simulink model "sgMdl_IO334_AnalogLoopbackOversampling"  (R2024b)
settings: Solver=FixedStepAuto  StartTime=0.0  StopTime=inf  RelTol=1e-3
undefined symbols (not defined in the file): AnalogOutputFrameSize, IO3xx, Pull, pull, SineFrequency, Ts, up
libraries: speedgoatlib_fpga_analog_io x3, slrealtimeloglib x2, simulink x1, speedgoatlib_interrupt x1, slrealtimetgmanagement x1, speedgoatlib_fpga x1
Description:
  | IO334 - Analog Loopback with Oversampling
settings Model: ModifiedByFormat=Speedgoat  SimulationMode=external  ExtModeTrigDuration=100000  Creator=Speedgoat  LastModifiedBy=Speedgoat
settings SolverCC: ConcurrentTasks=on  PositivePriorityOrder=on
settings DataIOCC: SaveFormat=StructureWithTime
settings OptimizationCC: BlockReduction=off  OptimizeBlockIOStorage=off  BufferReuse=off  ReuseModelBlockBuffer=off
settings DebuggingCC: UnderspecifiedInitializationDetection=Classic  MergeDetectMultiDrivingBlocksExec=none  TasksWithSamePriorityMsg=none
settings HardwareCC: ProdBitPerLong=64  ProdLongLongMode=on  ProdHWDeviceType=Intel->x86-64 (Linux 64)
settings ModelReferenceCC: EnableRefExpFcnMdlSchedulingChecks=on  PropagateSignalLabelsOutOfModel=off
settings RTWCC: Description=Speedgoat Real-Time Target Machine  SystemTargetFile=speedgoat.tlc  TemplateMakefile=slrealtime_default_tmf  PostCodeGenCommand=sg.model.build.makeCfg(bdroot, buildInfo);  Toolchain=Simulink Real-Time Toolchain  BuildConfiguration=Faster Runs  TargetLang=C++  GPUComputeCapability=3.5
settings SimulinkRealTimeTargetCC: SubcomponentCodeInterfacePackaging=Reusable function  InstructionSetFMA=off  LogToMDFFile=off  SLRTFileLogMaxRuns=10
settings ConfigComp: CovBoundaryAbsTol=1.0e-5

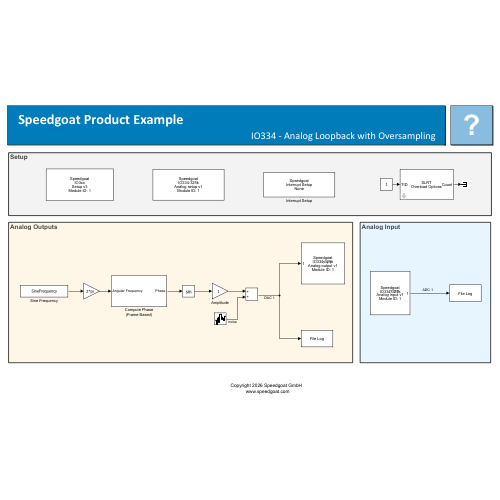
[thumbnail: Simulink's stored preview of the top-level diagram]
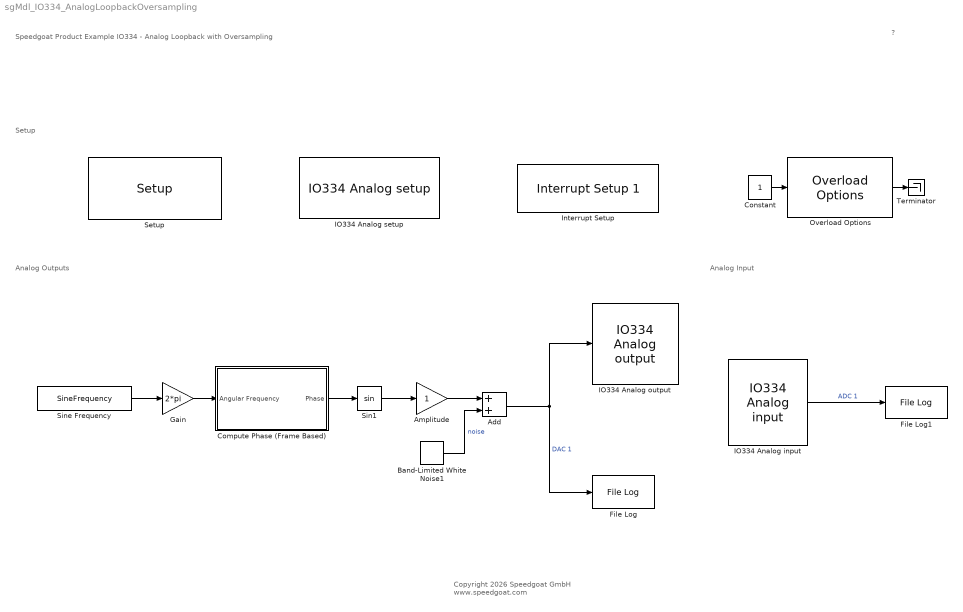
== system sgMdl_IO334_AnalogLoopbackOversampling ==
  note: Analog Outputs
  note: Analog Input
  note: Setup
  note: Speedgoat Product Example
      | IO334 - Analog Loopback with Oversampling
  note: ?
  note: Copyright 2026 Speedgoat GmbH
      |  www.speedgoat.com
  Add : Sum
  Amplitude : Gain
  Band-Limited White Noise1 : simulink/Sources/Band-Limited White Noise  Cov=[1e-6]  Ts=Ts  seed=round(rand(1,AnalogOutputFrameSize)*1000)
  Compute Phase (Frame Based) : Subsystem
  Constant : Constant  SampleTime=Ts
  File Log : slrealtimeloglib/File Log  decimation=1  inputProcessing=Columns as channels (frame based)
  File Log1 : slrealtimeloglib/File Log  decimation=1  inputProcessing=Elements as channels (sample based)
  Gain : Gain  Gain=2*pi
  IO334 Analog input : speedgoatlib_fpga_analog_io/IO334/IO334 Analog input  id=1  parSampleTime=-1  pciSlot=[-1,-1]  parAiChannels=1  parAiChannelsStreamed=1  parAiReadPrevValue=0  parAiEnableFrame=0  parAdcCoupling=[1 1 1 1]  parAdcContSampling=0  parAdcDmaEnable=0  parAdcActiveDmaDevices=[1 1 1 1]  parAiFrameSize=100
      settings: SourceProductName=Analog IO
  IO334 Analog output : speedgoatlib_fpga_analog_io/IO334/IO334 Analog output  id=1  parSampleTime=-1  pciSlot=[-1,-1]  board=Please select...  parAoChannels=1  parAoVoltageRange=1  parDacOverRange=[0 0 0 0 0 0 0 0]  parAoInitValues=0  parAoReset=0  parDacSyncOut=1  parAoEnableFrame=1  parDacActiveDmaDevices=[1 1 1 1]  parDacDmaLatency=2  parAoFrameSize=100
      settings: SourceProductName=Analog IO
  IO334 Analog setup : speedgoatlib_fpga_analog_io/IO334/IO334 Analog setup  id=1  parEnableCodeModule1=off  parEnableCodeModule2=off  parEnableCodeModule3=off  parEnableCodeModule4=off  parEnableCodeModule5=off  parEnableCodeModule6=off  parEnableCodeModule7=off  parEnableCodeModule8=off  parAdcEnableIndividualTrigger=off  parAdcDisableSampleRead=off  parAdcTriggerMode1=I/O Module Digital I/O  parAdcSampleRate1=1e6  parAdcDioTriggerChannel1=1  parAdcInternalTrigger1=<empty>  parAdcOversampling1=4  parAdcTriggerMode2=Model Step  parAdcSampleRate2=1e6  parAdcDioTriggerChannel2=1  parAdcInternalTrigger2=<empty>  parAdcOversampling2=4  parAdcTriggerMode3=I/O Module Digital I/O  parAdcSampleRate3=1e6  parAdcDioTriggerChannel3=1  parAdcInternalTrigger3=<empty>  parAdcOversampling3=4  parAdcTriggerMode4=I/O Module Internal Signal  parAdcSampleRate4=1e6  parAdcDioTriggerChannel4=1  parAdcInternalTrigger4=<empty>  parAdcOversampling4=4  parAdcTriggerMode5=I/O Module Clock  parAdcSampleRate5=1e6  parAdcDioTriggerChannel5=1  parAdcInternalTrigger5=<empty>  parAdcOversampling5=4  parAdcTriggerMode6=I/O Module Clock  parAdcSampleRate6=1e6  parAdcDioTriggerChannel6=1  parAdcInternalTrigger6=<empty>  parAdcOversampling6=4  parAdcTriggerMode7=I/O Module Clock  parAdcSampleRate7=1e6  parAdcDioTriggerChannel7=1  parAdcInternalTrigger7=<empty>  parAdcOversampling7=4  parAdcTriggerMode8=I/O Module Clock  parAdcSampleRate8=1e6  parAdcDioTriggerChannel8=1  parAdcInternalTrigger8=<empty>  parAdcOversampling8=4  parAdcReadPrevValueIndividualTrigger=off  parAdcEnableFrame=off  parAdcTriggerMode=I/O Module Clock  parAdcReadPrevValue=on  parAdcSampleRate=AnalogInputSampleRate  parAdcDioTriggerChannel=1  parAdcInternalTrigger=<empty>  parAdcOversampling=64  parAdcTriggerResolution=1e-08  parAdcSampleRateFrame=-1  parAdcFrameSize=100  parAdcSampleTime=Ts  parDacTriggerMode=I/O Module Clock  parDacInternalTrigger=<empty>  parDacDioTriggerChannel=1  parDacEnableFrame=on  dacUsesTimer=off  parDacFifoThreshold=AnalogOutputFrameSize*0.2  parDacTriggerResolution=1e-08  parDacSampleRate=-1  parDacFrameSize=AnalogOutputFrameSize  parDacSampleTime=Ts  parAdcChannel1=on  parAdcChannel2=off  parAdcChannel3=off  parAdcChannel4=off  parAdcChannel5=off  parAdcChannel6=off  parAdcChannel7=off  parAdcChannel8=off  parAdcChannel9=off  parAdcChannel10=off  parAdcChannel11=off  parAdcChannel12=off  parAdcChannel13=off  parAdcChannel14=off  parAdcChannel15=off  parAdcChannel16=off  parAdcAutoCorrection=on  parDacChannel1=on  parDacChannel2=off  parDacChannel3=off  parDacChannel4=off  parDacChannel5=off  parDacChannel6=off  parDacChannel7=off  parDacChannel8=off  parDacChannel9=off  parDacChannel10=off  parDacChannel11=off  parDacChannel12=off  parDacChannel13=off  parDacChannel14=off  parDacChannel15=off  parDacChannel16=off  parDacRange1=+-10 V  parDacInitValue1=0  parDacReset1=off  parDacRange2=+-5 V  parDacInitValue2=0  parDacReset2=off  parDacRange3=+-5 V  parDacInitValue3=0  parDacReset3=off  parDacRange4=+-5 V  parDacInitValue4=0  parDacReset4=off  parDacRange5=+-5 V  parDacInitValue5=0  parDacReset5=off  parDacRange6=+-5 V  parDacInitValue6=0  parDacReset6=off  parDacRange7=+-5 V  parDacInitValue7=0  parDacReset7=off  parDacRange8=+-5 V  parDacInitValue8=0  parDacReset8=off  parDacRange9=+-5 V  parDacInitValue9=0  parDacReset9=off  parDacRange10=+-5 V  parDacInitValue10=0  parDacReset10=off  parDacRange11=+-5 V  parDacInitValue11=0  parDacReset11=off  parDacRange12=+-5 V  parDacInitValue12=0  parDacReset12=off  parDacRange13=+-5 V  parDacInitValue13=0  parDacReset13=off  parDacRange14=+-5 V  parDacInitValue14=0  parDacReset14=off  parDacRange15=+-5 V  parDacInitValue15=0  parDacReset15=off  parDacRange16=+-5 V  parDacInitValue16=0  parDacReset16=off  parDacAutoCorrection=on
      settings: SourceProductName=Analog IO
  Interrupt Setup : speedgoatlib_interrupt/Interrupt Setup 1  parModuleTrigger=on  parPollingMode=on  parPriorityConf=High  parPriority=98  confStartFcn=IO334_325k_ANALOG_OUT_start_public  confStopFcn=IO334_325k_ANALOG_OUT_stop_public  confIsrFcn=IO334_325k_ANALOG_OUT_isr_public  confMapFcn=IO334_325k_ANALOG_OUT_map_public  confHookFile=io334_325k_analog_out_int_hooks.c  confIrqNr=-1  confIsPolling=on  confModID=16776961  confSelectedInt=Speedgoat IO334-325k Analog output interrupt  confSelectedId=1  confSelectedChannel=[]  confData=[90 1]  confForcePollingMode=off
  Overload Options : slrealtimetgmanagement/Overload Options  startupDur=1  startupDurSrc=Tunable Parameter  maxOverload=1  maxOverloadSrc=Tunable Parameter  TETFlag=off
  Setup : speedgoatlib_fpga/Setup/Setup  board=Please select...  id=1  pciSlot=-1  device_id=1  bitstreamFilePath=C:\SVN\speedgoatlib\releases\10.0.0\product_examples\IO334  bitstreamFile=Please select...  fpgaFreq=[100000000 125000000]  enableDma=on  rearEnb_1=off  rearIO_1=IO3xx-21  rearEnb_2=off  rearIO_2=None  ProgSpiFlash=off  ProgBPIFlash=off  useFpgaDmaController=off  dmaTrigDropdown=Model Step  dmaTrigSelect=0  dmaStopOnOverload=on  dmaModeSequential=on  dmaModeParallel=off  PullRPort15=pull-up 3.3V  PullRPort31=pull-up 3.3V  PullRPort47=pull-up 3.3V  PullRPort63=pull-up 3.3V  diffLineTermination_1=on  diffLineTermination_2=on  diffLineTermination_3=on  diffLineTermination_4=on  diffLineTermination_5=on  diffLineTermination_6=on  diffLineTermination_7=on  diffLineTermination_8=on  diffLineTermination_9=on  diffLineTermination_10=on  diffLineTermination_11=on  diffLineTermination_12=on  diffLineTermination_13=on  diffLineTermination_14=on  diffLineTermination_15=on  diffLineTermination_16=on  diffLineTermination_17=on  diffLineTermination_18=on  diffLineTermination_19=on  diffLineTermination_20=on  diffLineTermination_21=on  diffLineTermination_22=on  diffLineTermination_23=on  diffLineTermination_24=on  diffLineTermination_25=on  diffLineTermination_26=on  diffLineTermination_27=on  diffLineTermination_28=on  diffLineTermination_29=on  diffLineTermination_30=on  diffLineTermination_31=on  diffLineTermination_32=on  ioVoltageDropDown1=3.3V  pullResistorDropDown1_1=Pull-up  pullResistorDropDown1_2=Pull-up  pullResistorDropDown1_3=Pull-up  pullResistorDropDown1_4=Pull-up  pullResistorDropDown1_5=Pull-up  pullResistorDropDown1_6=Pull-up  pullResistorDropDown1_7=Pull-up  pullResistorDropDown1_8=Pull-up  ttlIsImplementedCheckBox1=off  pullResistorDropDown2=Pull-up  ioVoltageDropDown2=3.3V  ttlIsImplementedCheckBox2=off  pullResistorDropDown3=Pull-up  ioVoltageDropDown3=3.3V  ttlIsImplementedCheckBox3=off  pullResistorDropDown4=Pull-up  ioVoltageDropDown4=3.3V  ttlIsImplementedCheckBox4=off  pullResistorDropDown5=Pull-up  ioVoltageDropDown5=3.3V  ttlIsImplementedCheckBox5=off  pullResistorDropDown6=Pull-up  ioVoltageDropDown6=3.3V  ttlIsImplementedCheckBox6=off  pullResistorDropDown7=Pull-up  ioVoltageDropDown7=3.3V  ttlIsImplementedCheckBox7=off  pullResistorDropDown8=Pull-up  ioVoltageDropDown8=3.3V  ttlIsImplementedCheckBox8=off  terminationCheckBox1=off  terminationCheckBox2=off  terminationCheckBox3=off  terminationCheckBox4=off  diffIsImplementedCheckBox1=off  terminationCheckBox5=off  terminationCheckBox6=off  terminationCheckBox7=off  terminationCheckBox8=off  diffIsImplementedCheckBox2=off  terminationCheckBox9=off  terminationCheckBox10=off  terminationCheckBox11=off  terminationCheckBox12=off  diffIsImplementedCheckBox3=off  terminationCheckBox13=off  terminationCheckBox14=off  terminationCheckBox15=off  terminationCheckBox16=off  diffIsImplementedCheckBox4=off  terminationCheckBox17=off  terminationCheckBox18=off  terminationCheckBox19=off  terminationCheckBox20=off  diffIsImplementedCheckBox5=off  terminationCheckBox21=off  terminationCheckBox22=off  terminationCheckBox23=off  terminationCheckBox24=off  diffIsImplementedCheckBox6=off  terminationCheckBox25=off  terminationCheckBox26=off  terminationCheckBox27=off  terminationCheckBox28=off  diffIsImplementedCheckBox7=off  terminationCheckBox29=off  terminationCheckBox30=off  terminationCheckBox31=off  terminationCheckBox32=off  diffIsImplementedCheckBox8=off  PullRPort0_1=pull-up  VioPort0_1=3.3V  PullRPort1_1=pull-up  VioPort1_1=3.3V  PullRPort2_1=pull-up  VioPort2_1=3.3V  PullRPort3_1=pull-up  VioPort3_1=3.3V  PullRPort4_1=pull-up  VioPort4_1=3.3V  PullRPort5_1=pull-up  VioPort5_1=3.3V  PullRPort6_1=pull-up  VioPort6_1=3.3V  diffLineTermination_rear1_1=on  diffLineTermination_rear1_2=on  diffLineTermination_rear1_3=on  diffLineTermination_rear1_4=on  diffLineTermination_rear1_5=on  diffLineTermination_rear1_6=on  diffLineTermination_rear1_7=on  diffLineTermination_rear1_8=on  PullRPort0_2=pull-up  VioPort0_2=3.3V  PullRPort1_2=pull-up  VioPort1_2=3.3V  PullRPort2_2=pull-up  VioPort2_2=3.3V  PullRPort3_2=pull-up  VioPort3_2=3.3V  PullRPort4_2=pull-up  VioPort4_2=3.3V  PullRPort5_2=pull-up  VioPort5_2=3.3V  PullRPort6_2=pull-up  VioPort6_2=3.3V  diffLineTermination_rear2_1=on  diffLineTermination_rear2_2=on  diffLineTermination_rear2_3=on  diffLineTermination_rear2_4=on  diffLineTermination_rear2_5=on  diffLineTermination_rear2_6=on  diffLineTermination_rear2_7=on  diffLineTermination_rear2_8=on
      settings: SourceProductName=IO3xx
  Sin1 : Trigonometry
  Sine Frequency : Constant  Value=SineFrequency  SampleTime=Ts
  Terminator : Terminator
  wires:
  IO334 Analog input/1 -> File Log1/1  "ADC 1"
  Overload Options/1 -> Terminator/1
  Constant/1 -> Overload Options/1
  Gain/1 -> Compute Phase (Frame Based)/1(Angular Frequency)
  Sin1/1 -> Amplitude/1
  Amplitude/1 -> Add/1
  Add/1 -> IO334 Analog output/1, File Log/1  "DAC 1"
  Compute Phase (Frame Based)/1(Phase) -> Sin1/1
  Band-Limited White Noise1/1 -> Add/2  "noise"
  Sine Frequency/1 -> Gain/1

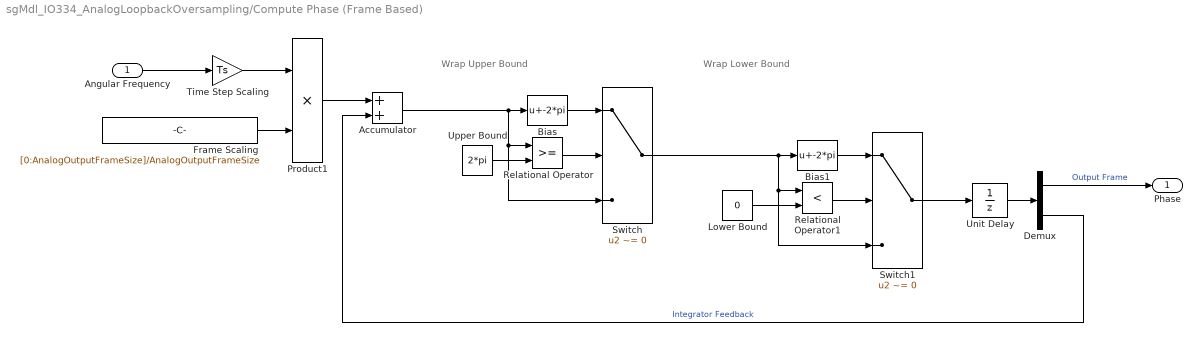
== system sgMdl_IO334_AnalogLoopbackOversampling/Compute Phase (Frame Based) ==
  note: Wrap Upper Bound
  note: Wrap Lower Bound
  Angular Frequency : Inport
  Accumulator : Sum
  Bias : Bias  Bias=-2*pi  SaturateOnIntegerOverflow=off
  Bias1 : Bias  Bias=-2*pi  SaturateOnIntegerOverflow=off
  Demux : Demux  Outputs=[AnalogOutputFrameSize,1]
  Frame Scaling : Constant  Value=[0:AnalogOutputFrameSize]/AnalogOutputFrameSize
  Lower Bound : Constant  Value=0
  Product1 : Product
  Relational Operator : RelationalOperator  OutDataTypeStr=boolean  RndMeth=Simplest  InputSameDT=off
  Relational Operator1 : RelationalOperator  Operator=<  OutDataTypeStr=boolean  RndMeth=Simplest  InputSameDT=off
  Switch : Switch  Criteria=u2 ~= 0  SaturateOnIntegerOverflow=off  InputSameDT=off
  Switch1 : Switch  Criteria=u2 ~= 0  SaturateOnIntegerOverflow=off  InputSameDT=off
  Time Step Scaling : Gain  Gain=Ts
  Unit Delay : UnitDelay  SampleTime=-1
  Upper Bound : Constant  Value=2*pi
  Phase : Outport
  wires:
  Angular Frequency/1 -> Time Step Scaling/1
  Accumulator/1 -> Bias/1, Switch/3, Relational Operator/1
  Upper Bound/1 -> Relational Operator/2
  Relational Operator/1 -> Switch/2
  Bias/1 -> Switch/1
  Bias1/1 -> Switch1/1
  Relational Operator1/1 -> Switch1/2
  Lower Bound/1 -> Relational Operator1/2
  Switch/1 -> Relational Operator1/1, Switch1/3, Bias1/1
  Switch1/1 -> Unit Delay/1
  Demux/2 -> Accumulator/2  "Integrator Feedback"
  Time Step Scaling/1 -> Product1/1
  Frame Scaling/1 -> Product1/2
  Product1/1 -> Accumulator/1
  Unit Delay/1 -> Demux/1
  Demux/1 -> Phase/1  "Output Frame"
